simulink model "Discrete_Equation"  (R2023a)
settings: Solver=VariableStepAuto  StartTime=0.0  StopTime=10.0  RelTol=1e-3
settings Model: Creator=Aman  LastModifiedBy=Aman

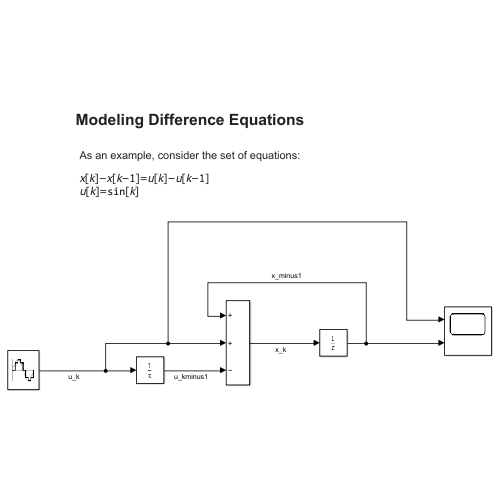
[thumbnail: Simulink's stored preview of the top-level diagram]
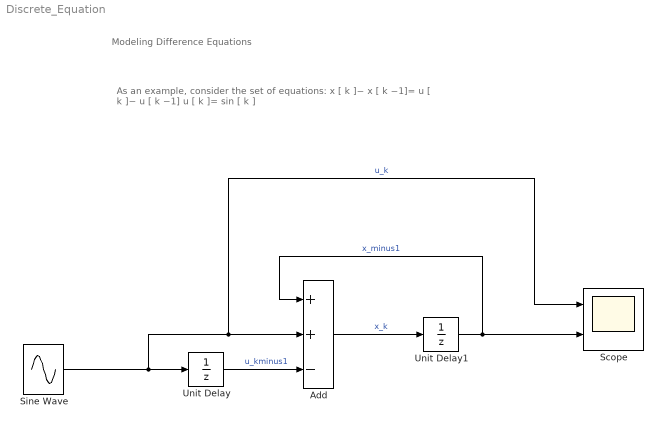
== system Discrete_Equation ==
  note: As an example, consider the set of equations:
      |
      | x [ k ]− x [ k −1]= u [ k ]− u [ k −1]
      | u [ k ]= sin [ k ]
  note: Modeling Difference Equations
  Add : Sum  Inputs=++-
  Scope : Scope  NumInputPorts=2
  Sine Wave : Sin  SampleTime=0.25
  Unit Delay : UnitDelay  InitialCondition=5  SampleTime=0.5  HasFrameUpgradeWarning=on
  Unit Delay1 : UnitDelay  InitialCondition=3  SampleTime=0.75  HasFrameUpgradeWarning=on
  wires:
  Sine Wave/1 -> Scope/1, Add/2, Unit Delay/1  "u_k"
  Unit Delay/1 -> Add/3  "u_kminus1"
  Add/1 -> Unit Delay1/1  "x_k"
  Unit Delay1/1 -> Scope/2, Add/1  "x_minus1"
